simulink model "svpwm"  (R2021a)
settings: Solver=VariableStepAuto  StartTime=0.0  StopTime=1  MaxStep=5e-6  RelTol=1e-3
undefined symbols (not defined in the file): fpm, fsw, iqmax, Lq, pp, Vdc
libraries: spsDiodeLib x6, spsIGBTLib x6, electricdrivelib x5, pid_lib x3, simulink x2, spsDCVoltageSourceLib x1, spsPermanentMagnetSynchronousMachineLib x1, simulink_extras x1, spsSawtoothGeneratorLib x1, spsSpaceVectorModulatorLib x1, mcbcontrolslib x1, spsTHDLib x1
settings Model: Creator=Ogün Altun  LastModifiedBy=enes_
settings SolverCC: ZeroCrossAlgorithm=Adaptive  AlgebraicLoopSolver=TrustRegion
settings DataIOCC: ReturnWorkspaceOutputs=off
settings DebuggingCC: MaxConsecutiveZCsMsg=none  SFMachineParentedDataDiag=warning  ArithmeticOperatorsInVariantConditions=warning
settings SFSimCC: SimUseLocalCustomCode=off  CustomCodeUndefinedFunction=UseInterfaceOnly
settings RTWCC: RTWUseLocalCustomCode=off

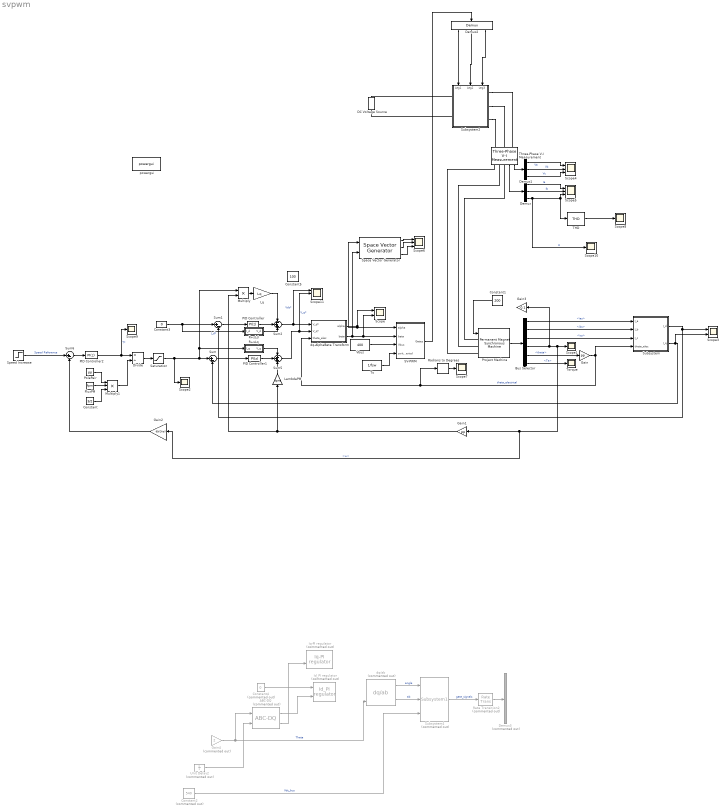
== system svpwm ==
  ABC-DQ : electricdrivelib/Fundamental Drive Blocks/Vector Controller (PMSM)/Detailed 3 phase SVM/ABC-DQ  Commented=on
      settings: SourceProductBaseCode=PS
  Bus Selector : BusSelector  OutputSignals=ias,ibs,ics,w,theta,Te
  Constant : Constant  Value=3/2
  Constant1 : Constant  Value=200
  Constant2 : Constant  Commented=on  Value=540
  Constant3 : Constant  Value=0
  Constant4 : Constant  Commented=on  Value=0
  Constant5 : Constant  Value=100
  DC Voltage Source : spsDCVoltageSourceLib/DC Voltage Source  Amplitude=Vdc  Measurements=None
  Demux : Demux  Outputs=3
  Demux1 : Demux  Outputs=3
  Demux2 : Demux  Outputs=3
  Demux3 : Demux  Commented=on  Outputs=6
  Divide : Product  Inputs=*/
  FluxPM : Constant  Value=fpm
  Gain : Gain  Gain=pp
  Gain1 : Gain  Gain=pp
  Gain2 : Gain  Gain=60/(2*pi)
  Gain3 : Gain  Gain=0.1
  Gain4 : Gain  Commented=on  Gain=2  SaturateOnIntegerOverflow=on  OutDataTypeStr=Inherit: Same as input  ParamDataTypeStr=Inherit: Same as input
  Id_PI regulator : electricdrivelib/Fundamental Drive Blocks/Vector Controller (PMSM)/Detailed 3 phase SVM/Id_PI regulator  Commented=on
      settings: SourceProductBaseCode=PS
  Iq-PI regulator : electricdrivelib/Fundamental Drive Blocks/Vector Controller (PMSM)/Detailed 3 phase SVM/Iq-PI regulator  Commented=on
      settings: SourceProductBaseCode=PS
  LambdaPM : Gain  Gain=fpm
  Lq : Gain  Gain=Lq
  Multiply : Product
  Multiply1 : Product  Inputs=3
  PID Controller : pid_lib/PID Controller  Controller=PI  Form=Parallel  TimeDomain=Discrete-time  UseExternalTs=off  SampleTime=-1  IntegratorMethod=Forward Euler  FilterMethod=Forward Euler  ControllerParametersSource=internal  P=1/10  I=250/10  D=0  UseFilter=on  N=100  TunerSelectOption=Transfer Function Based (PID Tuner App)  InitialConditionSource=internal  InitialConditionForIntegrator=0  InitialConditionForFilter=0  DifferentiatorICPrevScaledInput=0  ExternalReset=none  TrackingMode=off  Kt=1  LimitOutput=off  SatLimitsSource=internal  UpperSaturationLimit=inf  LowerSaturationLimit=-inf  LinearizeAsGain=on  AntiWindupMode=none  Kb=1  POutMin=[]  POutMax=[]  IOutMin=[]  IOutMax=[]  DOutMin=[]  DOutMax=[]  NOutMin=[]  NOutMax=[]  SumOutMin=[]  SumOutMax=[]  SaturationOutMin=[]  SaturationOutMax=[]  PParamMin=[]  PParamMax=[]  IParamMin=[]  IParamMax=[]  DParamMin=[]  DParamMax=[]  NParamMin=[]  NParamMax=[]  KbParamMin=[]  KbParamMax=[]  KtParamMin=[]  KtParamMax=[]  KbOutMin=[]  KbOutMax=[]  KtOutMin=[]  KtOutMax=[]  IntegratorOutMin=[]  IntegratorOutMax=[]  FilterOutMin=[]  FilterOutMax=[]  SumI1OutMin=[]  SumI1OutMax=[]  SumI2OutMin=[]  SumI2OutMax=[]  SumI3OutMin=[]  SumI3OutMax=[]  SumI4OutMin=[]  SumI4OutMax=[]  SumDOutMin=[]  SumDOutMax=[]  DifferentiatorOutMin=[]  DifferentiatorOutMax=[]  FilterDiffOutCoefMin=[]  FilterDiffOutCoefMax=[]  ReciprocalOutMin=[]  ReciprocalOutMax=[]  SumDenOutMin=[]  SumDenOutMax=[]  SumNumOutMin=[]  SumNumOutMax=[]  DivideOutMin=[]  DivideOutMax=[]  UdiffTsProdOutMin=[]  UdiffTsProdOutMax=[]  NTsProdOutMin=[]  NTsProdOutMax=[]  UintegralTsProdOutMin=[]  UintegralTsProdOutMax=[]  UngainTsProdOutMin=[]  UngainTsProdOutMax=[]  IntegratorContinuousStateAttributes=''  IntegratorStateMustResolveToSignalObject=off  IntegratorRTWStateStorageClass=Auto  FilterContinuousStateAttributes=''  FilterStateMustResolveToSignalObject=off  FilterRTWStateStorageClass=Auto  ParallelPVariant=InternalParameters  IdealPVariant=Disabled  IVariant=InternalParameters  DVariant=Disabled  IntegratorVariant=Discrete  SatVariant=Disabled  AWVariant=Passthrough  PCopyVariant=Disabled  TRVariant=Disabled  FdbkBlocksVariant=Forward  IdealPFdbkVariant=Disabled  SatFdbkVariant=Disabled  DerivativeFilterVariant=Disabled  NVariant=Disabled  NCopyVariant=Disabled_SignalSpec  FilterICVariant=Disabled  IntegratorICVariant=InternalICs  ExternalResetVariant=Disabled  TRSumVariant=Passthrough  SumFdbkVariant=Disabled  SumVariant=Sum_PI  TsampFilterVariant=InternalTs  TsampNgainVariant=Passthrough  TsampIntegralVariant=Passthrough  ExternalSaturationOutDataTypeStr=Inherit: Same as second input
  PID Controller1 : pid_lib/PID Controller  Controller=PI  Form=Parallel  TimeDomain=Discrete-time  UseExternalTs=off  SampleTime=-1  IntegratorMethod=Forward Euler  FilterMethod=Forward Euler  ControllerParametersSource=internal  P=1/10  I=250/10  D=0  UseFilter=on  N=100  TunerSelectOption=Transfer Function Based (PID Tuner App)  InitialConditionSource=internal  InitialConditionForIntegrator=0  InitialConditionForFilter=0  DifferentiatorICPrevScaledInput=0  ExternalReset=none  TrackingMode=off  Kt=1  LimitOutput=off  SatLimitsSource=internal  UpperSaturationLimit=inf  LowerSaturationLimit=-inf  LinearizeAsGain=on  AntiWindupMode=none  Kb=1  POutMin=[]  POutMax=[]  IOutMin=[]  IOutMax=[]  DOutMin=[]  DOutMax=[]  NOutMin=[]  NOutMax=[]  SumOutMin=[]  SumOutMax=[]  SaturationOutMin=[]  SaturationOutMax=[]  PParamMin=[]  PParamMax=[]  IParamMin=[]  IParamMax=[]  DParamMin=[]  DParamMax=[]  NParamMin=[]  NParamMax=[]  KbParamMin=[]  KbParamMax=[]  KtParamMin=[]  KtParamMax=[]  KbOutMin=[]  KbOutMax=[]  KtOutMin=[]  KtOutMax=[]  IntegratorOutMin=[]  IntegratorOutMax=[]  FilterOutMin=[]  FilterOutMax=[]  SumI1OutMin=[]  SumI1OutMax=[]  SumI2OutMin=[]  SumI2OutMax=[]  SumI3OutMin=[]  SumI3OutMax=[]  SumI4OutMin=[]  SumI4OutMax=[]  SumDOutMin=[]  SumDOutMax=[]  DifferentiatorOutMin=[]  DifferentiatorOutMax=[]  FilterDiffOutCoefMin=[]  FilterDiffOutCoefMax=[]  ReciprocalOutMin=[]  ReciprocalOutMax=[]  SumDenOutMin=[]  SumDenOutMax=[]  SumNumOutMin=[]  SumNumOutMax=[]  DivideOutMin=[]  DivideOutMax=[]  UdiffTsProdOutMin=[]  UdiffTsProdOutMax=[]  NTsProdOutMin=[]  NTsProdOutMax=[]  UintegralTsProdOutMin=[]  UintegralTsProdOutMax=[]  UngainTsProdOutMin=[]  UngainTsProdOutMax=[]  IntegratorContinuousStateAttributes=''  IntegratorStateMustResolveToSignalObject=off  IntegratorRTWStateStorageClass=Auto  FilterContinuousStateAttributes=''  FilterStateMustResolveToSignalObject=off  FilterRTWStateStorageClass=Auto  ParallelPVariant=InternalParameters  IdealPVariant=Disabled  IVariant=InternalParameters  DVariant=Disabled  IntegratorVariant=Discrete  SatVariant=Disabled  AWVariant=Passthrough  PCopyVariant=Disabled  TRVariant=Disabled  FdbkBlocksVariant=Forward  IdealPFdbkVariant=Disabled  SatFdbkVariant=Disabled  DerivativeFilterVariant=Disabled  NVariant=Disabled  NCopyVariant=Disabled_SignalSpec  FilterICVariant=Disabled  IntegratorICVariant=InternalICs  ExternalResetVariant=Disabled  TRSumVariant=Passthrough  SumFdbkVariant=Disabled  SumVariant=Sum_PI  TsampFilterVariant=InternalTs  TsampNgainVariant=Passthrough  TsampIntegralVariant=Passthrough  ExternalSaturationOutDataTypeStr=Inherit: Same as second input
  PID Controller2 : pid_lib/PID Controller  Controller=PI  Form=Parallel  TimeDomain=Discrete-time  UseExternalTs=off  SampleTime=-1  IntegratorMethod=Forward Euler  FilterMethod=Forward Euler  ControllerParametersSource=internal  P=1000  I=1  D=0  UseFilter=on  N=100  TunerSelectOption=Transfer Function Based (PID Tuner App)  InitialConditionSource=internal  InitialConditionForIntegrator=0  InitialConditionForFilter=0  DifferentiatorICPrevScaledInput=0  ExternalReset=none  TrackingMode=off  Kt=1  LimitOutput=off  SatLimitsSource=internal  UpperSaturationLimit=inf  LowerSaturationLimit=-inf  LinearizeAsGain=on  AntiWindupMode=none  Kb=1  POutMin=[]  POutMax=[]  IOutMin=[]  IOutMax=[]  DOutMin=[]  DOutMax=[]  NOutMin=[]  NOutMax=[]  SumOutMin=[]  SumOutMax=[]  SaturationOutMin=[]  SaturationOutMax=[]  PParamMin=[]  PParamMax=[]  IParamMin=[]  IParamMax=[]  DParamMin=[]  DParamMax=[]  NParamMin=[]  NParamMax=[]  KbParamMin=[]  KbParamMax=[]  KtParamMin=[]  KtParamMax=[]  KbOutMin=[]  KbOutMax=[]  KtOutMin=[]  KtOutMax=[]  IntegratorOutMin=[]  IntegratorOutMax=[]  FilterOutMin=[]  FilterOutMax=[]  SumI1OutMin=[]  SumI1OutMax=[]  SumI2OutMin=[]  SumI2OutMax=[]  SumI3OutMin=[]  SumI3OutMax=[]  SumI4OutMin=[]  SumI4OutMax=[]  SumDOutMin=[]  SumDOutMax=[]  DifferentiatorOutMin=[]  DifferentiatorOutMax=[]  FilterDiffOutCoefMin=[]  FilterDiffOutCoefMax=[]  ReciprocalOutMin=[]  ReciprocalOutMax=[]  SumDenOutMin=[]  SumDenOutMax=[]  SumNumOutMin=[]  SumNumOutMax=[]  DivideOutMin=[]  DivideOutMax=[]  UdiffTsProdOutMin=[]  UdiffTsProdOutMax=[]  NTsProdOutMin=[]  NTsProdOutMax=[]  UintegralTsProdOutMin=[]  UintegralTsProdOutMax=[]  UngainTsProdOutMin=[]  UngainTsProdOutMax=[]  IntegratorContinuousStateAttributes=''  IntegratorStateMustResolveToSignalObject=off  IntegratorRTWStateStorageClass=Auto  FilterContinuousStateAttributes=''  FilterStateMustResolveToSignalObject=off  FilterRTWStateStorageClass=Auto  ParallelPVariant=InternalParameters  IdealPVariant=Disabled  IVariant=InternalParameters  DVariant=Disabled  IntegratorVariant=Discrete  SatVariant=Disabled  AWVariant=Passthrough  PCopyVariant=Disabled  TRVariant=Disabled  FdbkBlocksVariant=Forward  IdealPFdbkVariant=Disabled  SatFdbkVariant=Disabled  DerivativeFilterVariant=Disabled  NVariant=Disabled  NCopyVariant=Disabled_SignalSpec  FilterICVariant=Disabled  IntegratorICVariant=InternalICs  ExternalResetVariant=Disabled  TRSumVariant=Passthrough  SumFdbkVariant=Disabled  SumVariant=Sum_PI  TsampFilterVariant=InternalTs  TsampNgainVariant=Passthrough  TsampIntegralVariant=Passthrough  ExternalSaturationOutDataTypeStr=Inherit: Same as second input
  PolePair : Constant  Value=pp
  Project Machine : spsPermanentMagnetSynchronousMachineLib/Permanent Magnet Synchronous Machine  NbPhases=3  FluxDistribution=Sinusoidal  RotorType=Round  MechanicalLoad=Torque Tm  PresetModel=No  ShowDetailedParameters=on  MeasurementBus=on  Resistance=1e-7  Inductance=8.5e-3  dqInductances=[8.5e-3,8.5e-3]  La=Lq  MachineConstant=Flux linkage established by magnets (V.s)  Flux=fpm  VoltageCst=52.2374  TorqueCst=0.432  Flat=120  Mechanical=[10 0 pp 0]  PolePairs=4  InitialConditions=[600, 0, 0,0]  InitialConditions5ph=[0 0 0 0 0 0]  RefAngle=Aligned with phase A axis (original Park)  IterativeDiscreteModel=Trapezoidal non iterative  TsBlock=-1  TsPowergui=0
  R+sLd : Subsystem
  R+sLq : Subsystem
  Radians to Degrees : simulink_extras/Transformations/Radians to Degrees
  Rate Transition2 : RateTransition  Commented=on
  SV-PWM : Subsystem
  Saturation : Saturate  UpperLimit=iqmax  LowerLimit=-iqmax
  Scope : Scope  NumInputPorts=2
  Scope{1..2,7..10} (6 alike) : Scope
  Scope{4..6,11} (4 alike) : Scope  NumInputPorts=3
  Scope3 : Scope  NumInputPorts=2
  Space Vector Generator : mcbcontrolslib/Space Vector Generator
      settings: SourceProductBaseCode=MT
  Speed Increase : Step  Time=0.5  Before=6000  After=6000  SampleTime=0
  Subsystem : Subsystem
  Subsystem2 : Subsystem
      settings: PortSchema="{\"entries\":[{\"content\":{\"sides\":[{\"content\":{\"connectorIds\":[\"LConn1\",\"LConn2\"]},\"type\":\"ConnectorPlacement.EquallySpacedRectSide\",\"uuid\":\"88d7e8af-40ab-4bee-bce0-34dcfd3f569e\"},{\"content\":{\"connectorIds\":[\"RConn1\",\"RConn2\",\"RConn3\"],\"side\":\"RIGHT\"},\"type\":\"ConnectorPlacement.EquallySpacedRectSide\",\"uuid\":\"521f4639-389b-4d4b-889c-c4a922300d9a\"},{\"content\":{\"connectorIds\":[\"In1\",\"In2\",\"In3\"],\"side\":\"TOP\"},\"type\":\"ConnectorPlacement.EquallySpacedRectSide\",\"uuid\":\"51a151b4-44d2-4df7-8739-c0682d747a60\"}]},\"type\":\"ConnectorPlacement.EquallySpacedConnector\",\"uuid\":\"fde39eeb-e449-4720-ab5d-3bded7fe6c71\"}],\"packageUris\":[\"http://schema.mathworks.com/mf0/Connector/R2020b\"],\"version\":\"1.0\"}"
  Subsystem4 : electricdrivelib/Fundamental Drive Blocks/Vector Controller (PMSM)/Detailed 3 phase SVM/Subsystem1  Commented=on  SystemSampleTime=-1
      settings: SourceProductBaseCode=PS
  Sum : Sum  Inputs=|+-
  Sum1 : Sum  Inputs=|+-
  Sum2 : Sum  Inputs=-++
  Sum5 : Sum  Inputs=+++
  Sum6 : Sum  Inputs=|+-
  THD : spsTHDLib/THD  Freq=50  Ts=0
      settings: SourceProductBaseCode=PS
  Three-Phase V-I Measurement : spsThreePhaseVIMeasurementLib/Three-Phase V-I Measurement  VoltageMeasurement=phase-to-phase  SetLabelV=off  LabelV=Vabc  Vpu=off  VpuLL=off  CurrentMeasurement=yes  SetLabelI=off  LabelI=Iabc  Ipu=off  Pbase=100e6  Vbase=500e3  OutputType=Complex  PhasorSimulation=off  PSBequivalent=0
  Torque : Scope
  Ts : Constant  Value=1/fsw
  Unit Delay2 : UnitDelay  Commented=on  SampleTime=-1  HasFrameUpgradeWarning=on
  Vbus : Constant  Value=400
  dq-AlphaBeta Transform : Subsystem
  dq/ab : electricdrivelib/Fundamental Drive Blocks/Vector Controller (PMSM)/Detailed 3 phase SVM/dq//ab  Commented=on  SystemSampleTime=-1
      settings: SourceProductBaseCode=PS
  powergui : spspowerguiLib/powergui  Priority=1  SimulationMode=Continuous  SampleTime=50e-6  frequency=60  Iterations=50  frequencyindice=0  Pbase=100e6  ErrMax=1e-4  UnitsV=kV  UnitsW=MW  buscounter=0  FunctionMessages=off  echomessages=off  EnableUseOfTLC=off  CurrentSourceSwitches=off  DisableSnubberDevices=off  DisableRonSwitches=off  DisableVfSwitches=off  DisplayEquations=off  AutomaticDiscreteSolvers=off  SolverType=Tustin/Backward Euler (TBE)  Interpol=off  ExternalGateDelay=off  methode=off  Ts=100  x0status=blocks  SPID=on  SwTol=0  HookPort=off  NonlinearTolerance=1e-4  nMaxIteration=100  ContinueOnMaxIteration=off  RestoreLinks=warning  ResistiveCurrentMeasurement=off  Frange=[0:2:500]  Ylog=off  Xlog=on  ShowGrid=off  save=off  variable=ZData  structure=ic_sine  ZoomFFT=off  StartTime=0.5  cycles=20  DisplayStyle=1  fundamental=50  FreqAxis=on  MaxFrequency=50*100  frequencyindicesteady=1  RmsSteady=1  display=off
  wires:
  Bus Selector/1 -> Subsystem/1(I_a)  "<ias>"
  Bus Selector/2 -> Subsystem/2(I_b)  "<ibs>"
  Bus Selector/3 -> Subsystem/3(I_c)  "<ics>"
  Bus Selector/4 -> Gain3/1, Scope1/1, Gain2/1, Gain1/1  "<w>"
  Bus Selector/5 -> Gain/1  "<theta>"
  Bus Selector/6 -> Torque/1  "<Te>"
  Gain/1 -> Radians to Degrees/1, dq-AlphaBeta Transform/3(theta_elec), Subsystem/4(theta_elec)  "theta_electrical"
  Sum/1 -> PID Controller1/1
  Sum1/1 -> PID Controller/1
  Subsystem/1(I_d) -> Sum1/2, Scope3/1
  Divide/1 -> Saturation/1
  Subsystem/2(I_q) -> Scope3/2, Sum/2
  PID Controller1/1 -> Sum5/2
  PID Controller/1 -> Sum2/2
  Gain2/1 -> Sum6/2
  Sum6/1 -> PID Controller2/1
  PID Controller2/1 -> Scope9/1, Divide/1  "T*"
  PolePair/1 -> Multiply1/1
  FluxPM/1 -> Multiply1/2
  Constant/1 -> Multiply1/3
  Multiply1/1 -> Divide/2
  Project Machine/1 -> Bus Selector/1
  Three-Phase V-I Measurement/1 -> Demux1/1
  Demux/1 -> Scope5/1  "Ia"
  Demux/2 -> Scope5/2  "Ib"
  Demux/3 -> Scope10/1, THD/1, Scope5/3  "Ic"
  Demux1/2 -> Scope4/2  "Vb"
  Demux1/1 -> Scope4/1  "Va"
  Demux1/3 -> Scope4/3  "Vc"
  Speed Increase/1 -> Sum6/1  "Speed Reference"
  Gain1/1 -> LambdaPM/1, Multiply/2
  R+sLd/1(V_d) -> Sum2/3
  R+sLq/1(V_q) -> Sum5/1
  Constant3/1 -> R+sLd/1(I_d), Sum1/1  "I_d*"
  Lq/1 -> Sum2/1
  LambdaPM/1 -> Sum5/3
  Multiply/1 -> Lq/1
  dq-AlphaBeta Transform/1("alpha ") -> Scope/1, SV-PWM/1(alpha), Space Vector Generator/1
  dq-AlphaBeta Transform/2(beta) -> SV-PWM/2(beta), Scope/2, Space Vector Generator/2
  Rate Transition2/1 -> Demux3/1
  Subsystem4/1 -> Rate Transition2/1  "gate_signals"
  Constant4/1 -> Id_PI regulator/1
  Three-Phase V-I Measurement/2 -> Demux/1
  Constant2/1 -> Subsystem4/3  "Vdc_bus"
  dq/ab/1 -> Subsystem4/1  "angle"
  Unit Delay2/1 -> ABC-DQ/2
  dq/ab/2 -> Subsystem4/2  "ab"
  Gain4/1 -> dq/ab/3, ABC-DQ/1  "Theta"
  ABC-DQ/2 -> Iq-PI regulator/2
  ABC-DQ/1 -> Id_PI regulator/2
  Saturation/1 -> Scope2/1, Multiply/1, R+sLq/1(I_q), Sum/1
  Radians to Degrees/1 -> Scope7/1
  Demux2/1 -> Subsystem2/1(Leg1)
  Demux2/2 -> Subsystem2/2(Leg2)
  Demux2/3 -> Subsystem2/3(Leg3)
  THD/1 -> Scope8/1
  SV-PWM/1(Gates) -> Demux2/1
  Ts/1 -> SV-PWM/4(switching period)
  Vbus/1 -> SV-PWM/3(Vbus)
  Constant1/1 -> Project Machine/1
  Sum2/1 -> Scope11/1, dq-AlphaBeta Transform/1(V_d*)  "Vds*"
  Sum5/1 -> Scope11/2, dq-AlphaBeta Transform/2(V_q*)  "V_q*"
  Space Vector Generator/1 -> Scope6/1
  Space Vector Generator/2 -> Scope6/2
  Space Vector Generator/3 -> Scope6/3
  connections:
  Subsystem2/LConn2 -- DC Voltage Source/LConn1
  Subsystem2/RConn1 -- Three-Phase V-I Measurement/LConn1
  Project Machine/LConn2 -- Three-Phase V-I Measurement/RConn2
  Project Machine/LConn3 -- Three-Phase V-I Measurement/RConn3
  Project Machine/LConn1 -- Three-Phase V-I Measurement/RConn1
  Subsystem2/RConn2 -- Three-Phase V-I Measurement/LConn2
  Subsystem2/RConn3 -- Three-Phase V-I Measurement/LConn3
  Subsystem2/LConn1 -- DC Voltage Source/RConn1

== system svpwm/R+sLd ==
  I_d : Inport
  Discrete Derivative : simulink/Discrete/Discrete Derivative  gainval=1.0  ICPrevScaledInput=0.0  OutMin=[]  OutMax=[]  OutDataType=fixdt(1, 16)  OutScaling=2^-10  DoSatur=off
  L : Gain  Gain=Lq
  V_d : Outport  VectorParamsAs1DForOutWhenUnconnected=off
  wires:
  I_d/1 -> L/1
  Discrete Derivative/1 -> V_d/1
  L/1 -> Discrete Derivative/1

== system svpwm/R+sLq ==
  I_q : Inport
  Discrete Derivative : simulink/Discrete/Discrete Derivative  gainval=1.0  ICPrevScaledInput=0.0  OutMin=[]  OutMax=[]  OutDataType=fixdt(1, 16)  OutScaling=2^-10  DoSatur=off
  L : Gain  Gain=Lq
  V_q : Outport  VectorParamsAs1DForOutWhenUnconnected=off
  wires:
  L/1 -> Discrete Derivative/1
  Discrete Derivative/1 -> V_q/1
  I_q/1 -> L/1

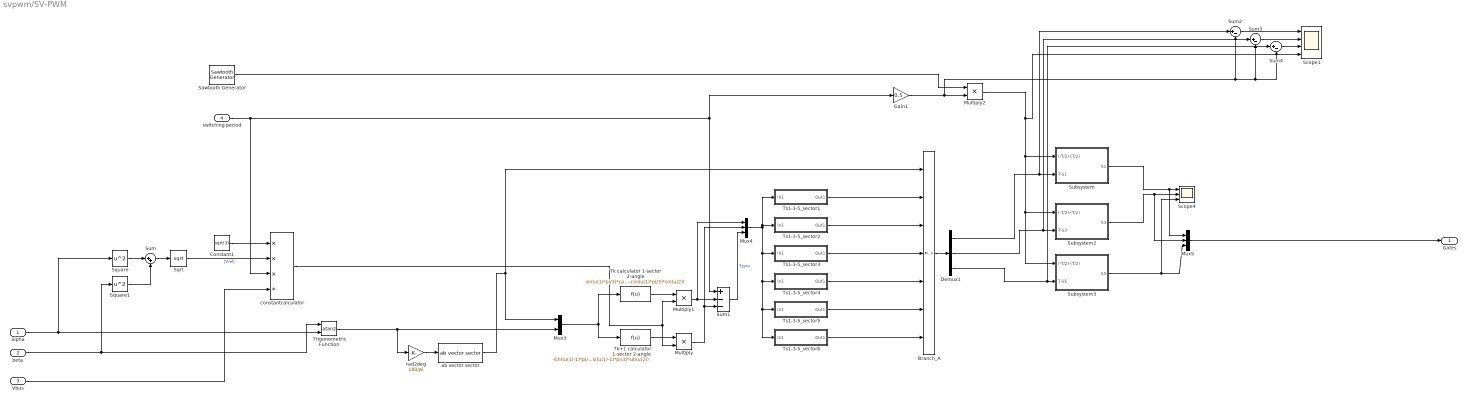
== system svpwm/SV-PWM ==
  alpha : Inport
  beta : Inport  Port=2
  Vbus : Inport  Port=3
  switching period : Inport  Port=4
  Branch_A : MultiPortSwitch  Inputs=6  SaturateOnIntegerOverflow=on  InputSameDT=on
  Constant1 : Constant  Value=sqrt(3)
  Demux1 : Demux  Outputs=3
  Gain1 : Gain  Gain=0.5
  Multiply : Product
  Multiply1 : Product
  Multiply2 : Product
  Mux3 : Mux  Inputs=2
  Mux4 : Mux  Inputs=3
  Mux5 : Mux  Inputs=3
  Sawtooth Generator : spsSawtoothGeneratorLib/Sawtooth Generator  Freq=10e3  Phase=180  Ts=0
  Scope1 : Scope  NumInputPorts=4
  Scope4 : Scope  NumInputPorts=3
  Sqrt : Sqrt  SaturateOnIntegerOverflow=on
  Square : Math  Operator=square  SignedPower=on  SaturateOnIntegerOverflow=on
  Square1 : Math  Operator=square  SignedPower=on  SaturateOnIntegerOverflow=on
  Subsystem : Subsystem
  Subsystem2 : Subsystem
  Subsystem3 : Subsystem
  Sum : Sum  Inputs=|++
  Sum1 : Sum  Inputs=+--
  Sum2 : Sum  Inputs=|+-
  Sum3 : Sum  Inputs=|+-
  Sum4 : Sum  Inputs=|+-
  Tk calculator 1-sector 2-angle : Fcn  Expr=sin(u(1)*pi/3)*cos(u(2))-cos(u(1)*pi/3)*sin(u(2))
  Tk+1 calculator 1-sector 2-angle : Fcn  Expr=-sin((u(1)-1)*pi/3)*cos(u(2))+cos((u(1)-1)*pi/3)*sin(u(2))
  Trigonometric Function : Trigonometry  Operator=atan2
  Ts1-3-5_sector1 : Subsystem
  Ts1-3-5_sector2 : Subsystem
  Ts1-3-5_sector3 : Subsystem
  Ts1-3-5_sector4 : Subsystem
  Ts1-3-5_sector5 : Subsystem
  Ts1-3-5_sector6 : Subsystem
  ab vector sector : spsSpaceVectorModulatorLib/Space Vector Modulator/Detailed/ab vector sector  SystemSampleTime=-1  VariantActivationTime=update diagram  Latency=0  AutoFrameSizeCalculation=off
      settings: SourceProductBaseCode=PS
  constantcalculator : Product  Inputs=***/
  rad2deg : Gain  Gain=180/pi  SaturateOnIntegerOverflow=on  OutDataTypeStr=Inherit: Same as input  ParamDataTypeStr=Inherit: Same as input
  Gates : Outport  VectorParamsAs1DForOutWhenUnconnected=off
  wires:
  rad2deg/1 -> ab vector sector/1
  Vbus/1 -> constantcalculator/4
  beta/1 -> Trigonometric Function/1, Square1/1
  Square/1 -> Sum/1
  Square1/1 -> Sum/2
  Sum/1 -> Sqrt/1
  Sqrt/1 -> constantcalculator/2  "|Vref|"
  Constant1/1 -> constantcalculator/1
  Mux3/1 -> Tk+1 calculator 1-sector 2-angle/1, Tk calculator 1-sector 2-angle/1
  switching period/1 -> constantcalculator/3, Gain1/1, Sum1/1
  Tk calculator 1-sector 2-angle/1 -> Multiply1/1
  Sum1/1 -> Mux4/3  "Tzero"
  Mux4/1 -> Ts1-3-5_sector2/1(In1), Ts1-3-5_sector1/1(In1), Ts1-3-5_sector4/1(In1), Ts1-3-5_sector6/1(In1), Ts1-3-5_sector5/1(In1), Ts1-3-5_sector3/1(In1)
  Ts1-3-5_sector1/1(Out1) -> Branch_A/2
  Ts1-3-5_sector2/1(Out1) -> Branch_A/3
  Ts1-3-5_sector3/1(Out1) -> Branch_A/4
  Ts1-3-5_sector4/1(Out1) -> Branch_A/5
  Ts1-3-5_sector5/1(Out1) -> Branch_A/6
  Ts1-3-5_sector6/1(Out1) -> Branch_A/7
  Branch_A/1 -> Demux1/1
  Demux1/1 -> Sum2/1, Subsystem/2(T-S1)
  Multiply2/1 -> Scope1/4, Subsystem3/1((-T/2)-(T/2)), Subsystem2/1((-T/2)-(T/2)), Subsystem/1((-T/2)-(T/2))
  Demux1/2 -> Sum3/1, Subsystem2/2(T-S3)
  Demux1/3 -> Sum4/1, Subsystem3/2(T-S5)
  Trigonometric Function/1 -> rad2deg/1, Mux3/2
  Tk+1 calculator 1-sector 2-angle/1 -> Multiply/1
  Multiply/1 -> Mux4/2, Sum1/3
  constantcalculator/1 -> Multiply/2, Multiply1/2
  Multiply1/1 -> Mux4/1, Sum1/2
  Subsystem/1(S1) -> Mux5/1, Scope4/1
  Subsystem2/1(S3) -> Mux5/2, Scope4/2
  Subsystem3/1(S5) -> Scope4/3, Mux5/3
  Mux5/1 -> Gates/1
  Sawtooth Generator/1 -> Multiply2/1
  ab vector sector/1 -> Branch_A/1, Mux3/1
  alpha/1 -> Square/1, Trigonometric Function/2
  Gain1/1 -> Sum4/2, Sum3/2, Sum2/2, Multiply2/2
  Sum4/1 -> Scope1/3
  Sum3/1 -> Scope1/2
  Sum2/1 -> Scope1/1

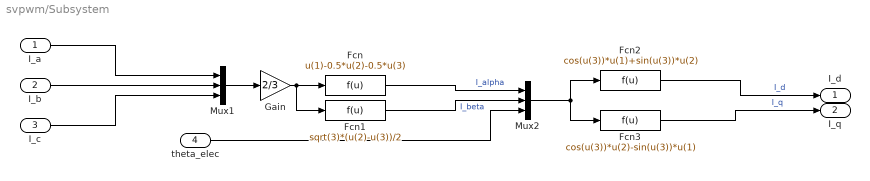
== system svpwm/Subsystem ==
  I_a : Inport
  I_b : Inport  Port=2
  I_c : Inport  Port=3
  theta_elec : Inport  Port=4
  Fcn : Fcn  Expr=u(1)-0.5*u(2)-0.5*u(3)
  Fcn1 : Fcn  Expr=sqrt(3)*(u(2)-u(3))/2
  Fcn2 : Fcn  Expr=cos(u(3))*u(1)+sin(u(3))*u(2)
  Fcn3 : Fcn  Expr=cos(u(3))*u(2)-sin(u(3))*u(1)
  Gain : Gain  Gain=2/3
  Mux1 : Mux  Inputs=3
  Mux2 : Mux  Inputs=3
  I_d : Outport  VectorParamsAs1DForOutWhenUnconnected=off
  I_q : Outport  Port=2  VectorParamsAs1DForOutWhenUnconnected=off
  wires:
  theta_elec/1 -> Mux2/3
  Fcn1/1 -> Mux2/2  "I_beta"
  Mux1/1 -> Gain/1
  Fcn/1 -> Mux2/1  "I_alpha"
  Mux2/1 -> Fcn3/1, Fcn2/1
  Fcn3/1 -> I_q/1  "I_q"
  I_b/1 -> Mux1/2
  I_a/1 -> Mux1/1
  Fcn2/1 -> I_d/1  "I_d"
  I_c/1 -> Mux1/3
  Gain/1 -> Fcn1/1, Fcn/1

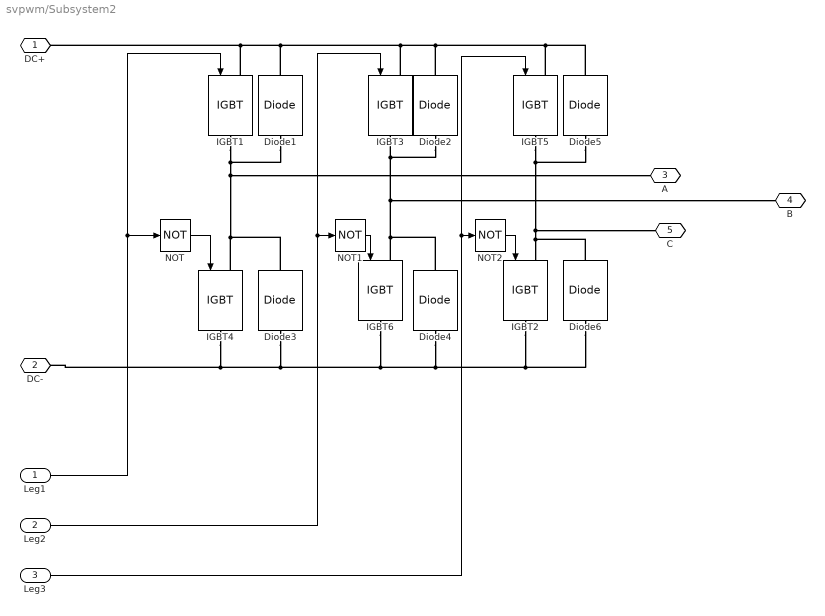
== system svpwm/Subsystem2 ==
  Leg1 : Inport
  Leg2 : Inport  Port=2
  Leg3 : Inport  Port=3
  Diode{1..6} (6 alike) : spsDiodeLib/Diode  Ron=0.0001  Lon=0  Vf=0  IC=0  UseSnubber=0  Rs=inf  Cs=0  Measurements=off
  IGBT{1..6} (6 alike) : spsIGBTLib/IGBT  Ron=0.001  Lon=0  Vf=0  Tf=1e-6  Tt=2e-6  IC=0  Rs=inf  Cs=inf  Measurements=off
  NOT : Logic  Operator=NOT  IconShape=distinctive  AllPortsSameDT=off  OutDataTypeStr=boolean
  NOT1 : Logic  Operator=NOT  IconShape=distinctive  AllPortsSameDT=off  OutDataTypeStr=boolean
  NOT2 : Logic  Operator=NOT  IconShape=distinctive  AllPortsSameDT=off  OutDataTypeStr=boolean
  DC+ : PMIOPort  Side=Left
  DC- : PMIOPort  Port=2  Side=Left
  A : PMIOPort  Port=3  Side=Right
  B : PMIOPort  Port=4  Side=Right
  C : PMIOPort  Port=5  Side=Right
  wires:
  NOT1/1 -> IGBT6/1
  Leg3/1 -> IGBT5/1, NOT2/1
  Leg2/1 -> NOT1/1, IGBT3/1
  Leg1/1 -> NOT/1, IGBT1/1
  NOT/1 -> IGBT4/1
  NOT2/1 -> IGBT2/1
  connections:
  IGBT5/RConn1 -- Diode5/LConn1 -- IGBT2/LConn1 -- Diode6/RConn1 -- C/RConn1
  IGBT4/LConn1 -- Diode3/RConn1 -- IGBT1/RConn1 -- Diode1/LConn1 -- A/RConn1
  Diode5/RConn1 -- IGBT5/LConn1 -- Diode2/RConn1 -- IGBT3/LConn1 -- Diode1/RConn1 -- DC+/RConn1 -- IGBT1/LConn1
  IGBT3/RConn1 -- IGBT6/LConn1 -- Diode4/RConn1 -- B/RConn1 -- Diode2/LConn1
  IGBT6/RConn1 -- Diode6/LConn1 -- IGBT2/RConn1 -- Diode4/LConn1 -- IGBT4/RConn1 -- DC-/RConn1 -- Diode3/LConn1

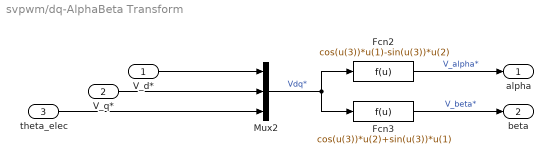
== system svpwm/dq-AlphaBeta Transform ==
  V_d* : Inport
  V_q* : Inport  Port=2
  theta_elec : Inport  Port=3
  Fcn2 : Fcn  Expr=cos(u(3))*u(1)-sin(u(3))*u(2)
  Fcn3 : Fcn  Expr=cos(u(3))*u(2)+sin(u(3))*u(1)
  Mux2 : Mux  Inputs=3
  "alpha " : Outport  VectorParamsAs1DForOutWhenUnconnected=off
  beta : Outport  Port=2  VectorParamsAs1DForOutWhenUnconnected=off
  wires:
  Mux2/1 -> Fcn2/1, Fcn3/1  "Vdq*"
  Fcn3/1 -> beta/1  "V_beta*"
  V_d*/1 -> Mux2/1
  Fcn2/1 -> "alpha "/1  "V_alpha*"
  theta_elec/1 -> Mux2/3
  V_q*/1 -> Mux2/2

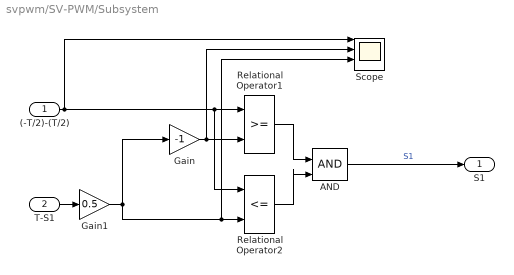
== system svpwm/SV-PWM/Subsystem ==
  (-T/2)-(T/2) : Inport
  T-S1 : Inport  Port=2
  AND : Logic  IconShape=distinctive  AllPortsSameDT=off  OutDataTypeStr=boolean
  Gain : Gain  Gain=-1
  Gain1 : Gain  Gain=0.5
  Relational Operator1 : RelationalOperator  OutDataTypeStr=boolean  RndMeth=Simplest
  Relational Operator2 : RelationalOperator  Operator=<=  OutDataTypeStr=boolean  RndMeth=Simplest
  Scope : Scope  NumInputPorts=4
  S1 : Outport  VectorParamsAs1DForOutWhenUnconnected=off
  wires:
  AND/1 -> S1/1  "S1"
  Relational Operator2/1 -> AND/2
  Gain1/1 -> Scope/3, Relational Operator2/2, Gain/1
  Relational Operator1/1 -> AND/1
  T-S1/1 -> Gain1/1
  Gain/1 -> Scope/2, Relational Operator1/2
  (-T/2)-(T/2)/1 -> Scope/1, Relational Operator2/1, Relational Operator1/1

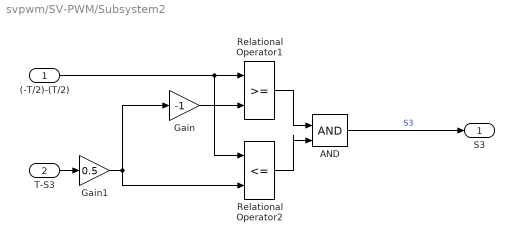
== system svpwm/SV-PWM/Subsystem2 ==
  (-T/2)-(T/2) : Inport
  T-S3 : Inport  Port=2
  AND : Logic  IconShape=distinctive  AllPortsSameDT=off  OutDataTypeStr=boolean
  Gain : Gain  Gain=-1
  Gain1 : Gain  Gain=0.5
  Relational Operator1 : RelationalOperator  OutDataTypeStr=boolean  RndMeth=Simplest
  Relational Operator2 : RelationalOperator  Operator=<=  OutDataTypeStr=boolean  RndMeth=Simplest
  S3 : Outport  VectorParamsAs1DForOutWhenUnconnected=off
  wires:
  Gain/1 -> Relational Operator1/2
  T-S3/1 -> Gain1/1
  Relational Operator1/1 -> AND/1
  Gain1/1 -> Gain/1, Relational Operator2/2
  (-T/2)-(T/2)/1 -> Relational Operator1/1, Relational Operator2/1
  Relational Operator2/1 -> AND/2
  AND/1 -> S3/1  "S3"

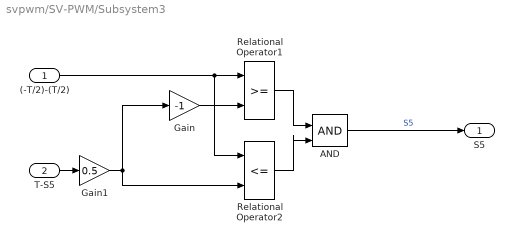
== system svpwm/SV-PWM/Subsystem3 ==
  (-T/2)-(T/2) : Inport
  T-S5 : Inport  Port=2
  AND : Logic  IconShape=distinctive  AllPortsSameDT=off  OutDataTypeStr=boolean
  Gain : Gain  Gain=-1
  Gain1 : Gain  Gain=0.5
  Relational Operator1 : RelationalOperator  OutDataTypeStr=boolean  RndMeth=Simplest
  Relational Operator2 : RelationalOperator  Operator=<=  OutDataTypeStr=boolean  RndMeth=Simplest
  S5 : Outport  VectorParamsAs1DForOutWhenUnconnected=off
  wires:
  AND/1 -> S5/1  "S5"
  Relational Operator2/1 -> AND/2
  (-T/2)-(T/2)/1 -> Relational Operator2/1, Relational Operator1/1
  Gain1/1 -> Relational Operator2/2, Gain/1
  Relational Operator1/1 -> AND/1
  T-S5/1 -> Gain1/1
  Gain/1 -> Relational Operator1/2

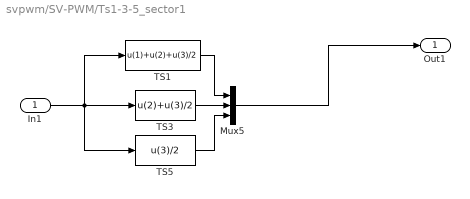
== system svpwm/SV-PWM/Ts1-3-5_sector1 ==
  In1 : Inport
  Mux5 : Mux  Inputs=3
  TS1 : Fcn  Expr=u(1)+u(2)+u(3)/2
  TS3 : Fcn  Expr=u(2)+u(3)/2
  TS5 : Fcn  Expr=u(3)/2
  Out1 : Outport  VectorParamsAs1DForOutWhenUnconnected=off
  wires:
  In1/1 -> TS3/1, TS5/1, TS1/1
  TS3/1 -> Mux5/2
  TS1/1 -> Mux5/1
  TS5/1 -> Mux5/3
  Mux5/1 -> Out1/1

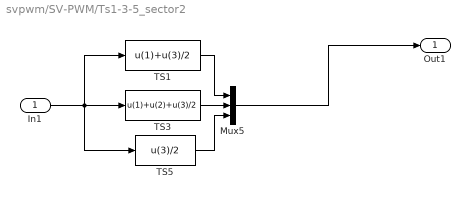
== system svpwm/SV-PWM/Ts1-3-5_sector2 ==
  In1 : Inport
  Mux5 : Mux  Inputs=3
  TS1 : Fcn  Expr=u(1)+u(3)/2
  TS3 : Fcn  Expr=u(1)+u(2)+u(3)/2
  TS5 : Fcn  Expr=u(3)/2
  Out1 : Outport  VectorParamsAs1DForOutWhenUnconnected=off
  wires:
  Mux5/1 -> Out1/1
  TS5/1 -> Mux5/3
  TS1/1 -> Mux5/1
  TS3/1 -> Mux5/2
  In1/1 -> TS1/1, TS5/1, TS3/1

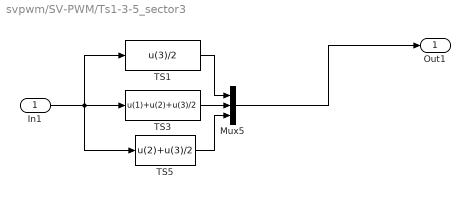
== system svpwm/SV-PWM/Ts1-3-5_sector3 ==
  In1 : Inport
  Mux5 : Mux  Inputs=3
  TS1 : Fcn  Expr=u(3)/2
  TS3 : Fcn  Expr=u(1)+u(2)+u(3)/2
  TS5 : Fcn  Expr=u(2)+u(3)/2
  Out1 : Outport  VectorParamsAs1DForOutWhenUnconnected=off
  wires:
  In1/1 -> TS3/1, TS5/1, TS1/1
  TS3/1 -> Mux5/2
  TS1/1 -> Mux5/1
  TS5/1 -> Mux5/3
  Mux5/1 -> Out1/1

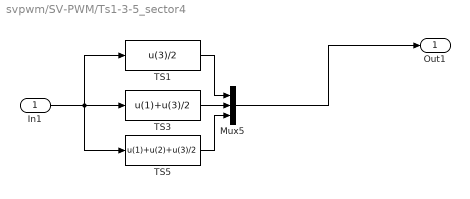
== system svpwm/SV-PWM/Ts1-3-5_sector4 ==
  In1 : Inport
  Mux5 : Mux  Inputs=3
  TS1 : Fcn  Expr=u(3)/2
  TS3 : Fcn  Expr=u(1)+u(3)/2
  TS5 : Fcn  Expr=u(1)+u(2)+u(3)/2
  Out1 : Outport  VectorParamsAs1DForOutWhenUnconnected=off
  wires:
  Mux5/1 -> Out1/1
  TS5/1 -> Mux5/3
  TS1/1 -> Mux5/1
  TS3/1 -> Mux5/2
  In1/1 -> TS1/1, TS5/1, TS3/1

== system svpwm/SV-PWM/Ts1-3-5_sector5 ==
  In1 : Inport
  Mux5 : Mux  Inputs=3
  TS1 : Fcn  Expr=u(2)+u(3)/2
  TS3 : Fcn  Expr=u(3)/2
  TS5 : Fcn  Expr=u(1)+u(2)+u(3)/2
  Out1 : Outport  VectorParamsAs1DForOutWhenUnconnected=off
  wires:
  In1/1 -> TS3/1, TS5/1, TS1/1
  TS3/1 -> Mux5/2
  TS1/1 -> Mux5/1
  TS5/1 -> Mux5/3
  Mux5/1 -> Out1/1

== system svpwm/SV-PWM/Ts1-3-5_sector6 ==
  In1 : Inport
  Mux5 : Mux  Inputs=3
  TS1 : Fcn  Expr=u(1)+u(2)+u(3)/2
  TS3 : Fcn  Expr=u(3)/2
  TS5 : Fcn  Expr=u(1)+u(3)/2
  Out1 : Outport  VectorParamsAs1DForOutWhenUnconnected=off
  wires:
  Mux5/1 -> Out1/1
  TS5/1 -> Mux5/3
  TS1/1 -> Mux5/1
  TS3/1 -> Mux5/2
  In1/1 -> TS1/1, TS5/1, TS3/1
